simulink model "KITTDynamics"  (R2016a)
settings: Solver=VariableStepAuto  StartTime=0.0  StopTime=8  MaxStep=0.01  RelTol=1e-3
values from neighbouring files (symbols this model uses):
  b = 0.0015    [KITTParameters.m]    (also in LIN.m = [(r12)^2-norm(x1)^2+norm(x2)^2; LINfor4.m = [(r12)^2-norm(x1)^2+norm(x2)^2; LINfor5.m = [ (r12)^2-norm(x1)^2+norm(x2)^2)
  c = getdata(find(strcmp('c:',getdata))+1)    [EPOfunctions.m]    (also in KITTParameters.m = 0.02)
  Famax = 80    [KITTParameters.m]
  m = 13    [KITTParameters.m]
settings Model: Creator=Joran  LastModifiedBy=Hendrik Jan
settings DataIOCC: LimitDataPoints=on
settings DebuggingCC: AllowSymbolicDim=off
settings ModelReferenceCC: PropagateSignalLabelsOutOfModel=off
settings GRTTargetCC: GeneratePreprocessorConditionals=Use local settings

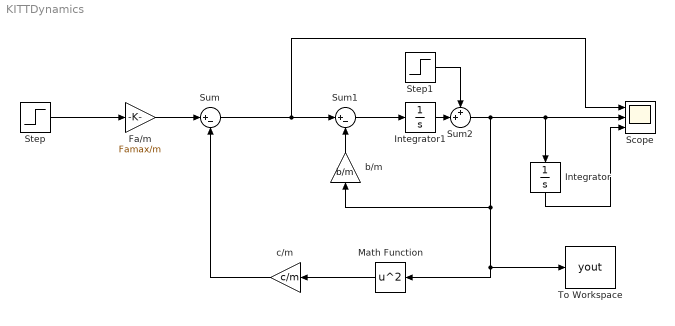
== system KITTDynamics ==
  Fa/m : Gain  Gain=Famax/m
  Integrator : Integrator
  Integrator1 : Integrator
  Math Function : Math  Operator=square  SaturateOnIntegerOverflow=on
  Scope : Scope  NumInputPorts=3
  Step : Step  SampleTime=0
  Step1 : Step  Time=0  Before=1  SampleTime=0
  Sum : Sum  Inputs=|+-
  Sum1 : Sum  Inputs=|+-
  Sum2 : Sum  Inputs=++|
  To Workspace : ToWorkspace  VariableName=yout  SaveFormat=Structure With Time  SampleTime=-1
      settings: Save2DSignal=2-D array (concatenate along first dimension)
  b/m : Gain  Gain=b/m
  c/m : Gain  Gain=c/m
  wires:
  Fa/m/1 -> Sum/1
  Sum1/1 -> Integrator1/1
  Step/1 -> Fa/m/1
  c/m/1 -> Sum/2
  b/m/1 -> Sum1/2
  Sum/1 -> Scope/1, Sum1/1
  Integrator/1 -> Scope/3
  Sum2/1 -> b/m/1, To Workspace/1, Math Function/1, Scope/2, Integrator/1
  Math Function/1 -> c/m/1
  Integrator1/1 -> Sum2/2
  Step1/1 -> Sum2/1
